simulink model "test_model_for_impedance_scan"  (R2020a)
settings: Solver=FixedStepDiscrete  StartTime=0.0  StopTime=1  FixedStep=1e-3  RelTol=1e-3
InitFcn:
  | Ts = 1e-3;
undefined symbols (not defined in the file or in its folder): freq
libraries: powerlib x15
settings Model: SimulationMode=accelerator  Creator=anony  LastModifiedBy=anony

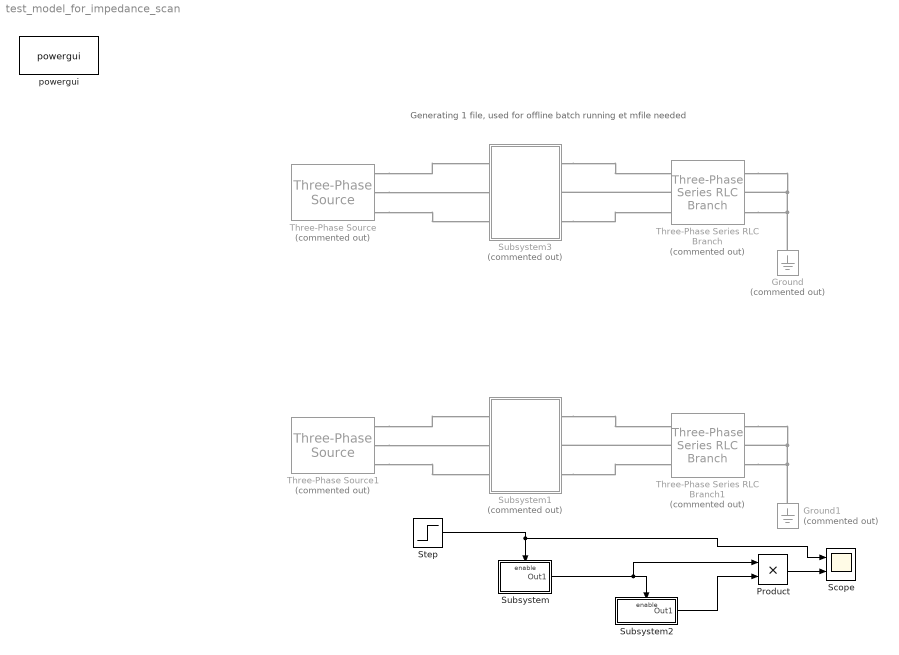
== system test_model_for_impedance_scan ==
  note: Generating 1 file, used for offline batch running et mfile needed
  Ground : powerlib/Elements/Ground  Commented=on  LConnTagsString=a
  Ground1 : powerlib/Elements/Ground  Commented=on  LConnTagsString=a
  Product : Product
  Scope : Scope  NumInputPorts=2
  Step : Step  Time=0.1  SampleTime=Ts
  Subsystem : Subsystem
  Subsystem1 : Subsystem  Commented=on  mask{t_start=1, frequency=freq, inject_duration=2, record_duration=1, stable_duration=1, amp_inject=35e3 * 0.02, t_Ts=Ts}
      mask prompts: t_start "启动时间 (s)"; frequency "待扫频率 (Hz)"; inject_duration "扰动时长 (s)"; record_duration "录波时长 (s)"; stable_duration "稳定时长 (s)"; amp_inject "扰动幅度 eg. 37e3 * 0.02"; t_Ts "Sample Ts"
  Subsystem2 : Subsystem
  Subsystem3 : Subsystem  Commented=on  mask{t_start=1, frequency=freq, inject_duration=2, record_duration=1, stable_duration=1, amp_inject=35e3 * 0.02, t_Ts=Ts}
      mask prompts: t_start "启动时间 (s)"; frequency "待扫频率 (Hz)"; inject_duration "扰动时长 (s)"; record_duration "录波时长 (s)"; stable_duration "稳定时长 (s)"; amp_inject "扰动幅度 eg. 37e3 * 0.02"; t_Ts "Sample Ts"
  Three-Phase Series RLC Branch : powerlib/Elements/Three-Phase Series RLC Branch  Commented=on  LConnTagsString=A|B|C  RConnTagsString=A|B|C  BranchType=RL  Resistance=1  Inductance=1e-2  Capacitance=1e-6  Measurements=None
  Three-Phase Series RLC Branch1 : powerlib/Elements/Three-Phase Series RLC Branch  Commented=on  LConnTagsString=A|B|C  RConnTagsString=A|B|C  BranchType=RL  Resistance=1  Inductance=1e-2  Capacitance=1e-6  Measurements=None
  Three-Phase Source : powerlib/Electrical Sources/Three-Phase Source  Commented=on  InternalConnection=Yg  VoltagePhases=off  Voltage=35e3  PhaseAngle=0  Voltage_phases=[25e3 25e3 25e3]/sqrt(3)  PhaseAngles_phases=[0 -120 +120]  Frequency=50  NonIdealSource=off  SpecifyImpedance=off  Resistance=0.8929  Inductance=16.58e-3  ShortCircuitLevel=100e6  BaseVoltage=25e3  XRratio=7  BusType=swing  Pref=10e3  Qref=0  Prefabc=[10e3, 10e3, 10e3]  Qrefabc=[0, 0, 0]  Qmin=-inf  Qmax=inf
  Three-Phase Source1 : powerlib/Electrical Sources/Three-Phase Source  Commented=on  InternalConnection=Yg  VoltagePhases=off  Voltage=35e3  PhaseAngle=0  Voltage_phases=[25e3 25e3 25e3]/sqrt(3)  PhaseAngles_phases=[0 -120 +120]  Frequency=50  NonIdealSource=off  SpecifyImpedance=off  Resistance=0.8929  Inductance=16.58e-3  ShortCircuitLevel=100e6  BaseVoltage=25e3  XRratio=7  BusType=swing  Pref=10e3  Qref=0  Prefabc=[10e3, 10e3, 10e3]  Qrefabc=[0, 0, 0]  Qmin=-inf  Qmax=inf
  powergui : powerlib/powergui  Priority=1  SimulationMode=Discrete  SampleTime=Ts  frequency=60  Iterations=50  frequencyindice=0  Pbase=100e6  ErrMax=1e-4  UnitsV=kV  UnitsW=MW  buscounter=0  FunctionMessages=off  echomessages=off  EnableUseOfTLC=off  CurrentSourceSwitches=off  DisableSnubberDevices=off  DisableRonSwitches=off  DisableVfSwitches=off  DisplayEquations=off  AutomaticDiscreteSolvers=off  SolverType=Tustin/Backward Euler (TBE)  Interpol=off  ExternalGateDelay=off  methode=off  Ts=100  x0status=blocks  SPID=on  SwTol=0  HookPort=off  NonlinearTolerance=1e-4  nMaxIteration=100  ContinueOnMaxIteration=off  RestoreLinks=warning  ResistiveCurrentMeasurement=off  Frange=[0:2:500]  Ylog=off  Xlog=on  ShowGrid=off  save=off  variable=ZData  structure=0  ZoomFFT=off  StartTime=0.0  cycles=1  DisplayStyle=1  fundamental=60  FreqAxis=off  MaxFrequency=1000  frequencyindicesteady=1  RmsSteady=1  display=off
  wires:
  Subsystem/1(Out1) -> Product/1, Subsystem2/Enable
  Step/1 -> Scope/1, Subsystem/Enable
  Subsystem2/1(Out1) -> Product/2
  Product/1 -> Scope/2
  connections:
  Ground/LConn1 -- Three-Phase Series RLC Branch/RConn3 -- Three-Phase Series RLC Branch/RConn1 -- Three-Phase Series RLC Branch/RConn2
  Three-Phase Source/RConn2 -- Subsystem3/LConn2
  Three-Phase Source/RConn1 -- Subsystem3/LConn1
  Three-Phase Source/RConn3 -- Subsystem3/LConn3
  Subsystem3/RConn1 -- Three-Phase Series RLC Branch/LConn1
  Three-Phase Series RLC Branch/LConn2 -- Subsystem3/RConn2
  Subsystem3/RConn3 -- Three-Phase Series RLC Branch/LConn3
  Ground1/LConn1 -- Three-Phase Series RLC Branch1/RConn2 -- Three-Phase Series RLC Branch1/RConn1 -- Three-Phase Series RLC Branch1/RConn3
  Three-Phase Series RLC Branch1/LConn2 -- Subsystem1/RConn2
  Three-Phase Source1/RConn3 -- Subsystem1/LConn3
  Subsystem1/RConn1 -- Three-Phase Series RLC Branch1/LConn1
  Three-Phase Source1/RConn2 -- Subsystem1/LConn2
  Three-Phase Source1/RConn1 -- Subsystem1/LConn1
  Subsystem1/RConn3 -- Three-Phase Series RLC Branch1/LConn3

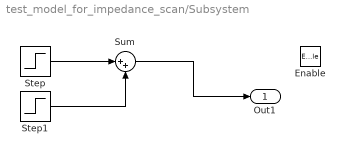
== system test_model_for_impedance_scan/Subsystem ==
  Enable : EnablePort
  Step : Step  Time=0  SampleTime=Ts
  Step1 : Step  Time=0.5  After=-1  SampleTime=Ts
  Sum : Sum  Inputs=|++
  Out1 : Outport
  wires:
  Sum/1 -> Out1/1
  Step/1 -> Sum/1
  Step1/1 -> Sum/2

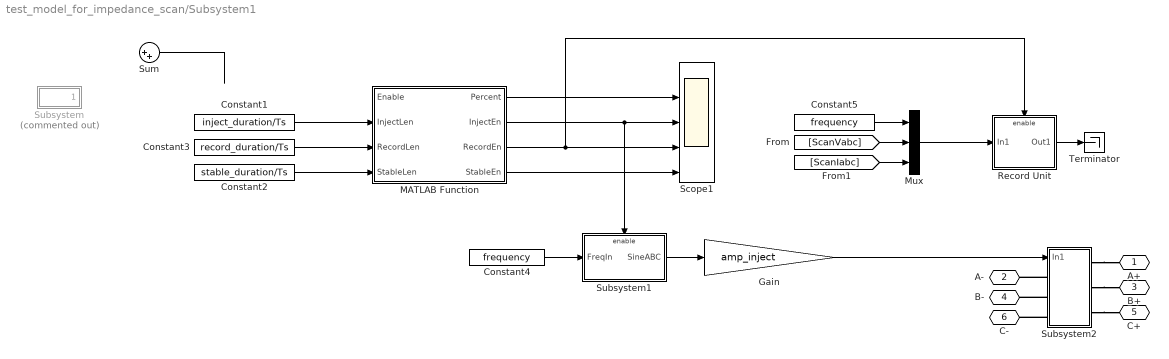
== system test_model_for_impedance_scan/Subsystem1 ==
  Constant1 : Constant  Value=inject_duration/Ts
  Constant2 : Constant  Value=stable_duration/Ts
  Constant3 : Constant  Value=record_duration/Ts
  Constant4 : Constant  Value=frequency
  Constant5 : Constant  Value=frequency
  Gain : Gain  Gain=amp_inject
  MATLAB Function : MATLAB Function  TreatAsAtomicUnit=on  SystemSampleTime=Ts
  Mux : Mux  Inputs=3
  Record Unit : Subsystem
  Scope1 : Scope  NumInputPorts=5
  Subsystem : Subsystem  Commented=on  mask{t_start=t_start, t_duration=inject_duration + stable_duration}
      mask prompts: t_start "Start Time"; t_duration "Duration"
  Subsystem1 : Subsystem
  Subsystem2 : Subsystem
  Sum : Sum  Inputs=|++
  Terminator : Terminator
  A+ : PMIOPort  Side=Right
  A- : PMIOPort  Port=2  Side=Left
  B+ : PMIOPort  Port=3  Side=Right
  B- : PMIOPort  Port=4  Side=Left
  C+ : PMIOPort  Port=5  Side=Right
  C- : PMIOPort  Port=6  Side=Left
  wires:
  Mux/1 -> Record Unit/1(In1)
  Gain/1 -> Subsystem2/1(In1)
  Subsystem1/1(SineABC) -> Gain/1
  [ScanVabc] -> Mux/2
  [ScanIabc] -> Mux/3
  Record Unit/1(Out1) -> Terminator/1
  Constant4/1 -> Subsystem1/1(FreqIn)
  MATLAB Function/4(StableEn) -> Scope1/5
  MATLAB Function/3(RecordEn) -> Scope1/4, Record Unit/Enable
  MATLAB Function/2(InjectEn) -> Scope1/3, Subsystem1/Enable
  Constant5/1 -> Mux/1
  Constant3/1 -> MATLAB Function/3(RecordLen)
  Constant2/1 -> MATLAB Function/4(StableLen)
  Constant1/1 -> MATLAB Function/2(InjectLen)
  MATLAB Function/1(Percent) -> Scope1/2
  ? -> MATLAB Function/1(Enable)
  Sum/1 -> ?
  connections:
  Subsystem2/RConn2 -- B+/RConn1
  Subsystem2/RConn1 -- A+/RConn1
  Subsystem2/LConn3 -- C-/RConn1
  Subsystem2/LConn2 -- B-/RConn1
  Subsystem2/LConn1 -- A-/RConn1
  Subsystem2/RConn3 -- C+/RConn1

== system test_model_for_impedance_scan/Subsystem2 ==
  Enable : EnablePort
  Pulse Generator : DiscretePulseGenerator  Period=10  PulseWidth=9  PhaseDelay=1  SampleTime=Ts
  Out1 : Outport
  wires:
  Pulse Generator/1 -> Out1/1

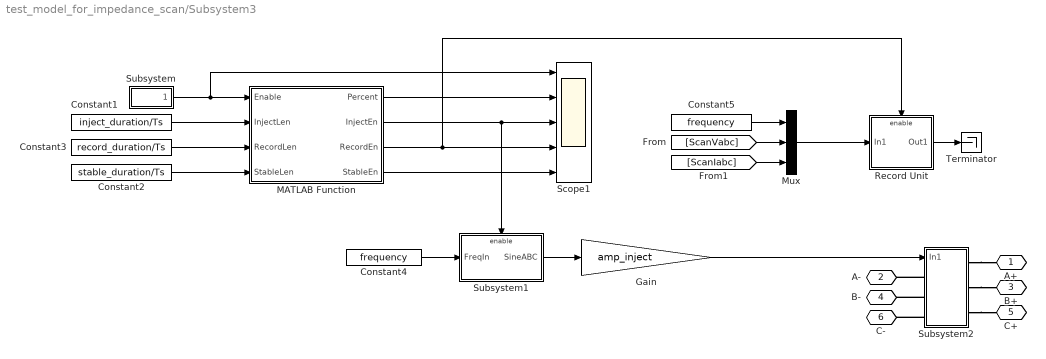
== system test_model_for_impedance_scan/Subsystem3 ==
  Constant1 : Constant  Value=inject_duration/Ts
  Constant2 : Constant  Value=stable_duration/Ts
  Constant3 : Constant  Value=record_duration/Ts
  Constant4 : Constant  Value=frequency
  Constant5 : Constant  Value=frequency
  Gain : Gain  Gain=amp_inject
  MATLAB Function : MATLAB Function  TreatAsAtomicUnit=on  SystemSampleTime=Ts
  Mux : Mux  Inputs=3
  Record Unit : Subsystem
  Scope1 : Scope  NumInputPorts=5
  Subsystem : Subsystem  mask{t_start=t_start, t_duration=inject_duration + stable_duration}
      mask prompts: t_start "Start Time"; t_duration "Duration"
  Subsystem1 : Subsystem
  Subsystem2 : Subsystem
  Terminator : Terminator
  A+ : PMIOPort  Side=Right
  A- : PMIOPort  Port=2  Side=Left
  B+ : PMIOPort  Port=3  Side=Right
  B- : PMIOPort  Port=4  Side=Left
  C+ : PMIOPort  Port=5  Side=Right
  C- : PMIOPort  Port=6  Side=Left
  wires:
  MATLAB Function/1(Percent) -> Scope1/2
  Subsystem/1(EnOut) -> Scope1/1, MATLAB Function/1(Enable)
  Constant1/1 -> MATLAB Function/2(InjectLen)
  Constant2/1 -> MATLAB Function/4(StableLen)
  Constant3/1 -> MATLAB Function/3(RecordLen)
  Constant5/1 -> Mux/1
  MATLAB Function/2(InjectEn) -> Subsystem1/Enable, Scope1/3
  MATLAB Function/3(RecordEn) -> Record Unit/Enable, Scope1/4
  MATLAB Function/4(StableEn) -> Scope1/5
  Constant4/1 -> Subsystem1/1(FreqIn)
  Record Unit/1(Out1) -> Terminator/1
  [ScanIabc] -> Mux/3
  [ScanVabc] -> Mux/2
  Subsystem1/1(SineABC) -> Gain/1
  Gain/1 -> Subsystem2/1(In1)
  Mux/1 -> Record Unit/1(In1)
  connections:
  Subsystem2/RConn3 -- C+/RConn1
  Subsystem2/LConn1 -- A-/RConn1
  Subsystem2/LConn2 -- B-/RConn1
  Subsystem2/LConn3 -- C-/RConn1
  Subsystem2/RConn1 -- A+/RConn1
  Subsystem2/RConn2 -- B+/RConn1

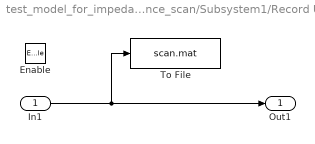
== system test_model_for_impedance_scan/Subsystem1/Record Unit ==
  In1 : Inport
  Enable : EnablePort
  To File : ToFile  Filename=scan.mat  MatrixName=scan  SampleTime=Ts
  Out1 : Outport
  wires:
  In1/1 -> Out1/1, To File/1

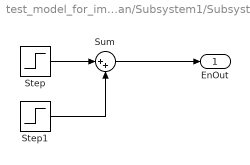
== system test_model_for_impedance_scan/Subsystem1/Subsystem ==
  Step : Step  Time=t_start  SampleTime=Ts
  Step1 : Step  Time=t_start+t_duration  After=-1  SampleTime=Ts
  Sum : Sum  Inputs=|++
  EnOut : Outport
  wires:
  Sum/1 -> EnOut/1
  Step/1 -> Sum/1
  Step1/1 -> Sum/2

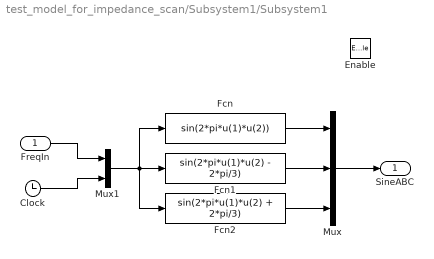
== system test_model_for_impedance_scan/Subsystem1/Subsystem1 ==
  FreqIn : Inport
  Enable : EnablePort
  Clock : Clock
  Fcn : Fcn  Expr=sin(2*pi*u(1)*u(2))
  Fcn1 : Fcn  Expr=sin(2*pi*u(1)*u(2) - 2*pi/3)
  Fcn2 : Fcn  Expr=sin(2*pi*u(1)*u(2) + 2*pi/3)
  Mux : Mux  Inputs=3
  Mux1 : Mux  Inputs=2
  SineABC : Outport
  wires:
  Fcn1/1 -> Mux/2
  Fcn/1 -> Mux/1
  Fcn2/1 -> Mux/3
  Mux/1 -> SineABC/1
  Mux1/1 -> Fcn2/1, Fcn/1, Fcn1/1
  FreqIn/1 -> Mux1/1
  Clock/1 -> Mux1/2

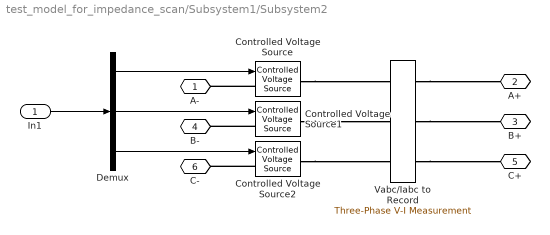
== system test_model_for_impedance_scan/Subsystem1/Subsystem2 ==
  In1 : Inport
  Controlled Voltage Source : powerlib/Electrical Sources/Controlled Voltage Source  Initialize=on  Source_Type=AC  Amplitude=0  Phase=0  Frequency=0  Measurements=None
  Controlled Voltage Source1 : powerlib/Electrical Sources/Controlled Voltage Source  Initialize=on  Source_Type=AC  Amplitude=0  Phase=0  Frequency=0  Measurements=None
  Controlled Voltage Source2 : powerlib/Electrical Sources/Controlled Voltage Source  Initialize=on  Source_Type=AC  Amplitude=0  Phase=0  Frequency=0  Measurements=None
  Demux : Demux  Outputs=3
  Vabc/Iabc to Record : powerlib/Measurements/Three-Phase V-I Measurement  VoltageMeasurement=phase-to-ground  SetLabelV=on  LabelV=ScanVabc  Vpu=off  VpuLL=off  CurrentMeasurement=yes  SetLabelI=on  LabelI=ScanIabc  Ipu=off  Pbase=100e6  Vbase=500e3  OutputType=Complex  PhasorSimulation=off  PSBequivalent=0
  A- : PMIOPort  Side=Left
  A+ : PMIOPort  Port=2  Side=Right
  B+ : PMIOPort  Port=3  Side=Right
  B- : PMIOPort  Port=4  Side=Left
  C+ : PMIOPort  Port=5  Side=Right
  C- : PMIOPort  Port=6  Side=Left
  wires:
  Demux/3 -> Controlled Voltage Source2/1
  Demux/2 -> Controlled Voltage Source1/1
  Demux/1 -> Controlled Voltage Source/1
  In1/1 -> Demux/1
  connections:
  Vabc/Iabc to Record/RConn1 -- A+/RConn1
  Controlled Voltage Source/RConn1 -- Vabc/Iabc to Record/LConn1
  Controlled Voltage Source1/RConn1 -- Vabc/Iabc to Record/LConn2
  Controlled Voltage Source2/RConn1 -- Vabc/Iabc to Record/LConn3
  Vabc/Iabc to Record/RConn3 -- C+/RConn1
  Controlled Voltage Source/LConn1 -- A-/RConn1
  Controlled Voltage Source1/LConn1 -- B-/RConn1
  Vabc/Iabc to Record/RConn2 -- B+/RConn1
  Controlled Voltage Source2/LConn1 -- C-/RConn1

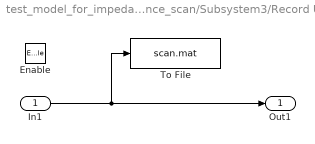
== system test_model_for_impedance_scan/Subsystem3/Record Unit ==
  In1 : Inport
  Enable : EnablePort
  To File : ToFile  Filename=scan.mat  MatrixName=scan  SampleTime=Ts
  Out1 : Outport
  wires:
  In1/1 -> To File/1, Out1/1

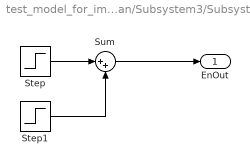
== system test_model_for_impedance_scan/Subsystem3/Subsystem ==
  Step : Step  Time=t_start  SampleTime=Ts
  Step1 : Step  Time=t_start+t_duration  After=-1  SampleTime=Ts
  Sum : Sum  Inputs=|++
  EnOut : Outport
  wires:
  Step1/1 -> Sum/2
  Step/1 -> Sum/1
  Sum/1 -> EnOut/1

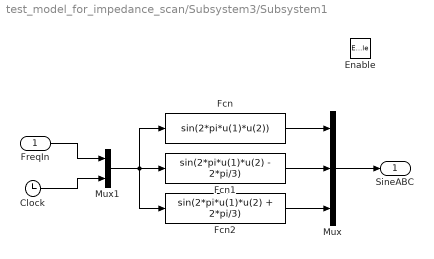
== system test_model_for_impedance_scan/Subsystem3/Subsystem1 ==
  FreqIn : Inport
  Enable : EnablePort
  Clock : Clock
  Fcn : Fcn  Expr=sin(2*pi*u(1)*u(2))
  Fcn1 : Fcn  Expr=sin(2*pi*u(1)*u(2) - 2*pi/3)
  Fcn2 : Fcn  Expr=sin(2*pi*u(1)*u(2) + 2*pi/3)
  Mux : Mux  Inputs=3
  Mux1 : Mux  Inputs=2
  SineABC : Outport
  wires:
  Clock/1 -> Mux1/2
  FreqIn/1 -> Mux1/1
  Mux1/1 -> Fcn1/1, Fcn/1, Fcn2/1
  Mux/1 -> SineABC/1
  Fcn2/1 -> Mux/3
  Fcn/1 -> Mux/1
  Fcn1/1 -> Mux/2

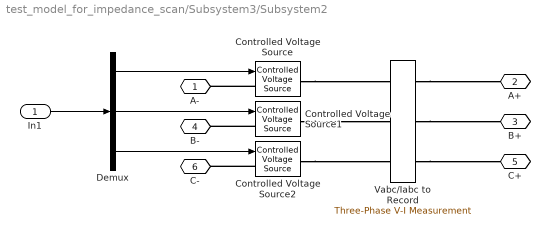
== system test_model_for_impedance_scan/Subsystem3/Subsystem2 ==
  In1 : Inport
  Controlled Voltage Source : powerlib/Electrical Sources/Controlled Voltage Source  Initialize=on  Source_Type=AC  Amplitude=0  Phase=0  Frequency=0  Measurements=None
  Controlled Voltage Source1 : powerlib/Electrical Sources/Controlled Voltage Source  Initialize=on  Source_Type=AC  Amplitude=0  Phase=0  Frequency=0  Measurements=None
  Controlled Voltage Source2 : powerlib/Electrical Sources/Controlled Voltage Source  Initialize=on  Source_Type=AC  Amplitude=0  Phase=0  Frequency=0  Measurements=None
  Demux : Demux  Outputs=3
  Vabc/Iabc to Record : powerlib/Measurements/Three-Phase V-I Measurement  VoltageMeasurement=phase-to-ground  SetLabelV=on  LabelV=ScanVabc  Vpu=off  VpuLL=off  CurrentMeasurement=yes  SetLabelI=on  LabelI=ScanIabc  Ipu=off  Pbase=100e6  Vbase=500e3  OutputType=Complex  PhasorSimulation=off  PSBequivalent=0
  A- : PMIOPort  Side=Left
  A+ : PMIOPort  Port=2  Side=Right
  B+ : PMIOPort  Port=3  Side=Right
  B- : PMIOPort  Port=4  Side=Left
  C+ : PMIOPort  Port=5  Side=Right
  C- : PMIOPort  Port=6  Side=Left
  wires:
  In1/1 -> Demux/1
  Demux/1 -> Controlled Voltage Source/1
  Demux/2 -> Controlled Voltage Source1/1
  Demux/3 -> Controlled Voltage Source2/1
  connections:
  Controlled Voltage Source2/LConn1 -- C-/RConn1
  Vabc/Iabc to Record/RConn2 -- B+/RConn1
  Controlled Voltage Source1/LConn1 -- B-/RConn1
  Controlled Voltage Source/LConn1 -- A-/RConn1
  Vabc/Iabc to Record/RConn3 -- C+/RConn1
  Controlled Voltage Source2/RConn1 -- Vabc/Iabc to Record/LConn3
  Controlled Voltage Source1/RConn1 -- Vabc/Iabc to Record/LConn2
  Controlled Voltage Source/RConn1 -- Vabc/Iabc to Record/LConn1
  Vabc/Iabc to Record/RConn1 -- A+/RConn1

== matlab function test_model_for_impedance_scan/Subsystem1/MATLAB Function ==
  data: Percent output; Enable input; InjectLen input; RecordLen input; StableLen input; InjectEn output; RecordEn output; StableEn output
function [Percent, InjectEn, RecordEn, StableEn] = fcn(Enable, InjectLen, RecordLen, StableLen)

persistent cnt_idx;
if isempty(cnt_idx)
    cnt_idx = 0;
    InjectEn = 0;
    RecordEn = 0;
    StableEn = 0;
else
    if Enable == 1
        if cnt_idx > 0 && cnt_idx <= (InjectLen-RecordLen)
            InjectEn = 1;
            RecordEn = 0;
            StableEn = 0;
        elseif cnt_idx > (InjectLen-RecordLen) && cnt_idx <= InjectLen
            InjectEn = 1;
            RecordEn = 1;
            StableEn = 0;
        elseif cnt_idx > InjectLen && cnt_idx <= (InjectLen + StableLen)
            InjectEn = 0;
            RecordEn = 0;
            StableEn = 1;
        else
            InjectEn = 0;
            RecordEn = 0;
            StableEn = 0;
        end
        cnt_idx = cnt_idx + 1;
    else
        cnt_idx = 0;
        InjectEn = 0;
        RecordEn = 0;
        StableEn = 0;
    end
end

Percent = cnt_idx;

== matlab function test_model_for_impedance_scan/Subsystem3/MATLAB Function ==
  data: Percent output; Enable input; InjectLen input; RecordLen input; StableLen input; InjectEn output; RecordEn output; StableEn output
function [Percent, InjectEn, RecordEn, StableEn] = fcn(Enable, InjectLen, RecordLen, StableLen)

persistent cnt_idx;
if isempty(cnt_idx)
    cnt_idx = 0;
    InjectEn = 0;
    RecordEn = 0;
    StableEn = 0;
else
    if Enable == 1
        if cnt_idx > 0 && cnt_idx <= (InjectLen-RecordLen)
            InjectEn = 1;
            RecordEn = 0;
            StableEn = 0;
        elseif cnt_idx > (InjectLen-RecordLen) && cnt_idx <= InjectLen
            InjectEn = 1;
            RecordEn = 1;
            StableEn = 0;
        elseif cnt_idx > InjectLen && cnt_idx <= (InjectLen + StableLen)
            InjectEn = 0;
            RecordEn = 0;
            StableEn = 1;
        else
            InjectEn = 0;
            RecordEn = 0;
            StableEn = 0;
        end
        cnt_idx = cnt_idx + 1;
    else
        cnt_idx = 0;
        InjectEn = 0;
        RecordEn = 0;
        StableEn = 0;
    end
end

Percent = cnt_idx;
